simulink model "CommSysSimulink"  (R2025b)
settings: Solver=VariableStepAuto  StartTime=0.0  StopTime=1  RelTol=1e-3
model workspace (MAT data in the model file):
  iSNR = 1
  x = 0
undefined symbols (not defined in the file): alpha, filterLenSymbols, modOrder, samplesPerSymbol, SNR, symRate
libraries: commdigbbndpm3 x6, commfilt2 x2, commdigbbndam3 x2, commchan3 x1, commsink2 x1, commseqgen3 x1, commrandsrc3 x1, simulink x1, commsync2 x1
settings Model: Creator=flora  LastModifiedBy=linnh

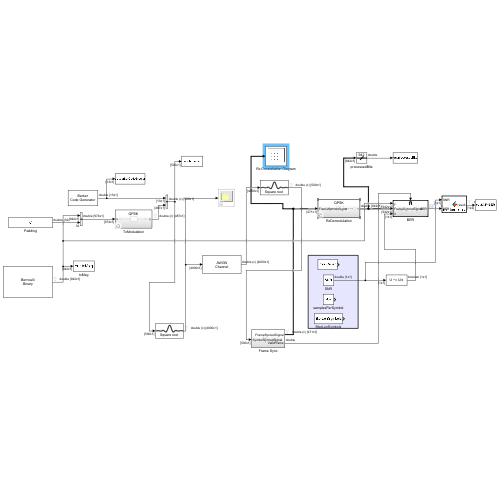
[thumbnail: Simulink's stored preview of the top-level diagram]
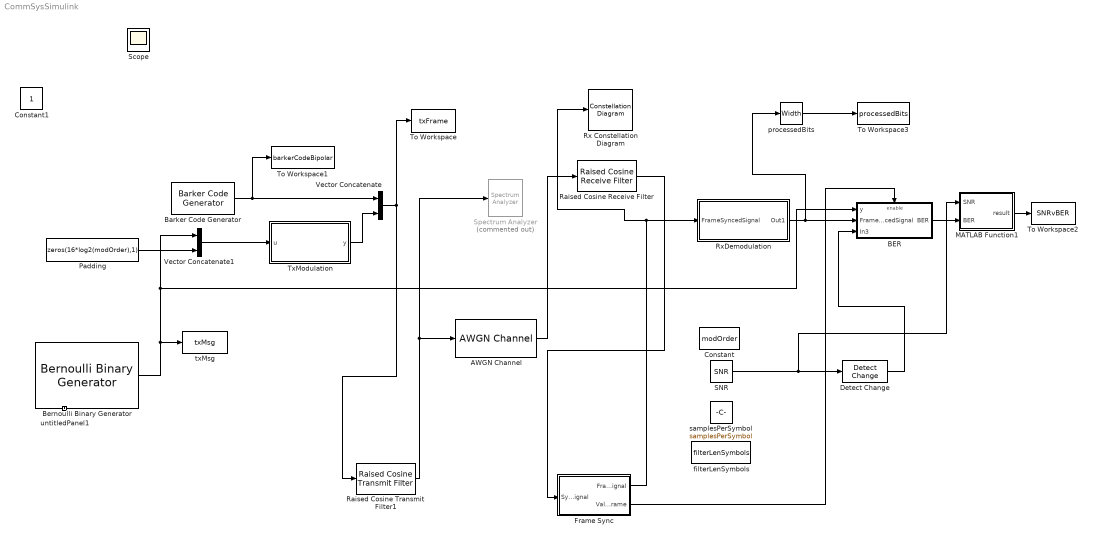
== system CommSysSimulink ==
  AWGN Channel : commchan3/AWGN Channel  LegacyMode=off  NoiseMethod="Signal to noise ratio  (Eb/No)"  noiseMode="Signal to noise ratio  (SNR)"  EbNo=SNR  EsNo=10  SNR=SNR  BitsPerSymbol=log2(modOrder)  SignalPower=1/samplesPerSymbol  SpecifySymbolPeriod=off  SamplesPerSymbol=samplesPerSymbol  SymbolPeriod=1  VarianceSource=Parameter  Variance=SNR/2  RandomStream=Global stream  Seed=67  SimulateUsing=Interpreted execution
  BER : Subsystem  TreatAsAtomicUnit=on
  Barker Code Generator : commseqgen3/Barker Code Generator  Length=7  LengthSimulink=13  SampleTime=-1  SamplesPerFrame=13  OutputDataType=double  SimulateUsing=Interpreted execution
  Bernoulli Binary Generator : commrandsrc3/Bernoulli Binary Generator  ProbabilityOfZero=0.5  SeedSource=Auto  Seed=0  SampleTime=1/(symRate*log2(modOrder))  SamplesPerFrame="(symRate  - 13 -16) * log2(modOrder)"  OutputDataType=double  SimulateUsing=Interpreted execution
  Constant : Constant  Value=modOrder
  Detect Change : simulink/Logic and Bit Operations/Detect Change  vinit=0  OutDataTypeStr=boolean
  Frame Sync : Subsystem
  MATLAB Function1 : MATLAB Function  TreatAsAtomicUnit=on
  Padding : Constant  Value=zeros(16*log2(modOrder),1)  SampleTime=-1
  Raised Cosine Receive Filter : commfilt2/Raised Cosine Receive Filter  filtType=Square root  R=alpha  filtSpan=10  N=8  downFactor=8  downOffset=0  filterGain=1  InputProcessing=Columns as channels (frame based)  RateOptions=Enforce single-rate processing  framing=Mute  checkCoeff=on  variableName=rcRxFilt  currentFiltSpan=10  D=5  inputOffset=0  sampMode=Mute  saveAsFlag=0  rateMode=Downsampling  checkGain=Normalized  launchFVT=on  roundingMode=Floor  overflowMode=off  coeffDataTypeStr=Inherit: Same word length as input  coeffMin=[]  coeffMax=[]  coeffLastDataTypeStr=Inherit: Same word length as input  accumDataTypeStr=Inherit: Same as product output  accumLastDataTypeStr=Inherit: Same as product output  outputDataTypeStr=Inherit: Same as accumulator  outputMin=[]  outputMax=[]  outputLastDataTypeStr=Inherit: Same as accumulator
  Raised Cosine Transmit Filter1 : commfilt2/Raised Cosine Transmit Filter  filtType=Square root  R=alpha  filtSpan=10  N=8  filterGain=1  InputProcessing=Columns as channels (frame based)  RateOptions=Enforce single-rate processing  framing=Mute  checkCoeff=on  variableName=rcTxFilt1  checkGain=Normalized  sampMode=Mute  saveAsFlag=0  currentFiltSpan=10  D=(10)/2  launchFVT=on  roundingMode=Floor  overflowMode=off  coeffDataTypeStr=Inherit: Same word length as input  coeffMin=[]  coeffMax=[]  coeffLastDataTypeStr=Inherit: Same word length as input  outputDataTypeStr=Inherit: Same as accumulator  outputMin=[]  outputMax=[]  outputLastDataTypeStr=Inherit: Same as accumulator
  Rx Constellation Diagram : ConstellationDiagram  WindowPosition=[320.000000,105.000000,737.000000,703.000000,]  Visible=on  ScopeFrameLocation=window  SymbolsToDisplay=100  ReferenceConstellation=BPSK  XLimits=[-2.68,2.53]  YLimits=[-2.68,2.53]  AxesLimits=[-2.68,2.53]  ShowReferenceConstellation=off
  RxDemodulation : Subsystem  Variant=on
  SNR : Constant  Value=SNR  VectorParams1D=off
  Spectrum Analyzer : SpectrumAnalyzer  Commented=on  WindowPosition=[589.000000,16.000000,654.000000,620.000000,]  ScopeFrameLocation=window  PlotAsTwoSidedSpectrum=off  Span=399999.99999999994  StartFrequency=-199999.99999999997  StopFrequency=199999.99999999997  YLimits=[-62.6319 17.8917]  ExpandToolstrip=on  SelectedToolstripTab=spectrumAnalyzerToolstrip.estimationTab
  To Workspace : ToWorkspace  VariableName=txFrame  SampleTime=-1
      settings: Save2DSignal=2-D array (concatenate along first dimension)
  To Workspace1 : ToWorkspace  VariableName=barkerCodeBipolar  SampleTime=-1
      settings: Save2DSignal=2-D array (concatenate along first dimension)
  To Workspace2 : ToWorkspace  VariableName=SNRvBER  SampleTime=-1
  To Workspace3 : ToWorkspace  VariableName=processedBits  SaveFormat=Timeseries  SampleTime=-1
  TxModulation : Subsystem  Variant=on
  Vector Concatenate : Concatenate
  Vector Concatenate1 : Concatenate
  filterLenSymbols : Constant  Value=filterLenSymbols
  processedBits : Width
  samplesPerSymbol : Constant  Value=samplesPerSymbol
  txMsg : ToWorkspace  VariableName=txMsg  SampleTime=-1
      settings: Save2DSignal=2-D array (concatenate along first dimension)
  untitledPanel1 : Subsystem  Tag=HiddenForWebPanel  IsWebBlockPanel=on
  Constant1 : Constant  IOType=siggen
  Scope : Scope
      settings: ActiveDisplayYMinimum=0.49969  ActiveDisplayYMaximum=0.49987
  wires:
  BER/1(BER) -> MATLAB Function1/2(BER)
  processedBits/1 -> To Workspace3/1
  Detect Change/1 -> BER/3(In3)
  Padding/1 -> Vector Concatenate1/2
  MATLAB Function1/1(result) -> To Workspace2/1
  TxModulation/1(y) -> Vector Concatenate/2
  Barker Code Generator/1 -> Vector Concatenate/1, To Workspace1/1
  SNR/1 -> Detect Change/1, MATLAB Function1/1(SNR)
  Bernoulli Binary Generator/1 -> txMsg/1, BER/1(y), Vector Concatenate1/1
  Vector Concatenate1/1 -> TxModulation/1(u)
  Vector Concatenate/1 -> Raised Cosine Transmit Filter1/1, To Workspace/1
  Raised Cosine Transmit Filter1/1 -> AWGN Channel/1, Spectrum Analyzer/1
  AWGN Channel/1 -> Raised Cosine Receive Filter/1
  Raised Cosine Receive Filter/1 -> Frame Sync/1(SymbolSyncedSignal)
  RxDemodulation/1(Out1) -> BER/2(FrameSyncedSignal), processedBits/1
  Frame Sync/1(FrameSyncedSignal) -> Rx Constellation Diagram/1, RxDemodulation/1(FrameSyncedSignal)
  Frame Sync/2(ValidFrame) -> BER/Enable

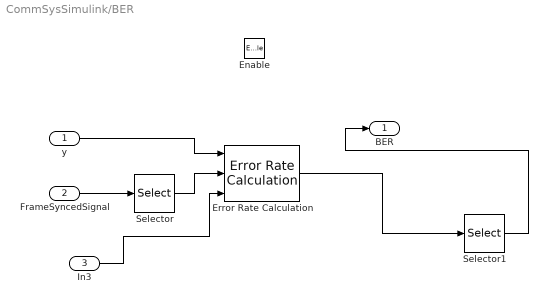
== system CommSysSimulink/BER ==
  y : Inport
  FrameSyncedSignal : Inport  Port=2
  In3 : Inport  Port=3
  Enable : EnablePort  PropagateVarSize=During execution
  Error Rate Calculation : commsink2/Error Rate Calculation  N=0  st_delay=0  cp_mode=Entire frame  subframe=[]  PMode=Port  WsName=ErrorVec  RsMode2=on  stop=off  numErr=100  maxBits=1e6
      settings: LibrarySourceBlock=|
      | commhdlsink/Error Rate
      | Calculation
  Selector : Selector  IndexOptions=Starting index (dialog)  Indices=1  OutputSizes="(symRate  - 13 -16) * log2(modOrder)"
  Selector1 : Selector  InputPortWidth=3  IndexOptions=Index vector (dialog)  Indices=1  OutputSizes=1
  BER : Outport
  wires:
  y/1 -> Error Rate Calculation/1
  Selector/1 -> Error Rate Calculation/2
  Error Rate Calculation/1 -> Selector1/1
  Selector1/1 -> BER/1
  FrameSyncedSignal/1 -> Selector/1
  In3/1 -> Error Rate Calculation/3

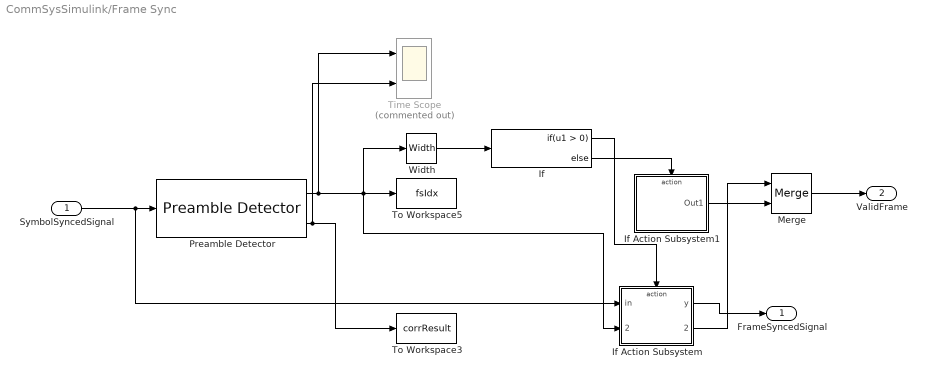
== system CommSysSimulink/Frame Sync ==
  SymbolSyncedSignal : Inport
  If : If
  If Action Subsystem : Subsystem  TreatAsAtomicUnit=on
  If Action Subsystem1 : Subsystem  TreatAsAtomicUnit=on
  Merge : Merge
  Preamble Detector : commsync2/Preamble Detector  Input=Symbol  Preamble=[-1;-1;-1;-1;-1;1;1;-1;-1;1;-1;1;-1]  Threshold=10  DetectionMetricOutput=on  Detections=First  SimulateUsing=Interpreted execution
  Time Scope : Scope  Commented=on  NumInputPorts=2
      settings: TimeUnits=Metric (based on Time Span)  Title=Preamble Detector Output  ActiveDisplayYMinimum=0  ActiveDisplayYMaximum=25  YLabel=Amplitude
  To Workspace3 : ToWorkspace  VariableName=corrResult  SaveFormat=Timeseries  SampleTime=-1
      settings: Save2DSignal=2-D array (concatenate along first dimension)
  To Workspace5 : ToWorkspace  VariableName=fsIdx  SaveFormat=Structure  SampleTime=-1
  Width : Width
  FrameSyncedSignal : Outport
  ValidFrame : Outport  Port=2
  wires:
  If Action Subsystem/1(y) -> FrameSyncedSignal/1
  Merge/1 -> ValidFrame/1
  Width/1 -> If/1
  Preamble Detector/2 -> To Workspace3/1, Time Scope/2
  If/1 -> If Action Subsystem/Action
  Preamble Detector/1 -> If Action Subsystem/2(peakIdx), To Workspace5/1, Width/1, Time Scope/1
  If Action Subsystem1/1(Out1) -> Merge/2
  If/2 -> If Action Subsystem1/Action
  SymbolSyncedSignal/1 -> Preamble Detector/1, If Action Subsystem/1(in)
  If Action Subsystem/2(ValidFrame) -> Merge/1

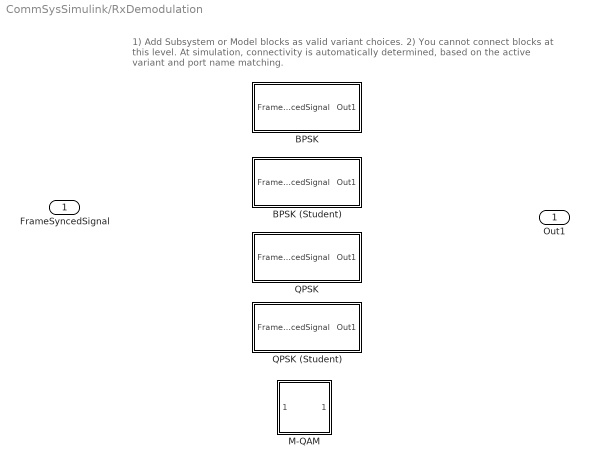
== system CommSysSimulink/RxDemodulation ==
  note: 1) Add Subsystem or Model blocks as valid variant choices.
      | 2) You cannot connect blocks at this level. At simulation, connectivity is automatically
      | determined, based on the active variant and port name matching.
  FrameSyncedSignal : Inport
  BPSK : Subsystem  VariantControl="modScheme==\"BPSK\""
  BPSK (Student) : Subsystem  VariantControl="modScheme==\"BPSK (Student)\""
  M-QAM : Subsystem  VariantControl="modScheme==\"M-QAM\""
  QPSK : Subsystem  VariantControl="modScheme==\"QPSK\""
  QPSK (Student) : Subsystem  VariantControl="modScheme==\"QPSK (Student)\""
  Out1 : Outport

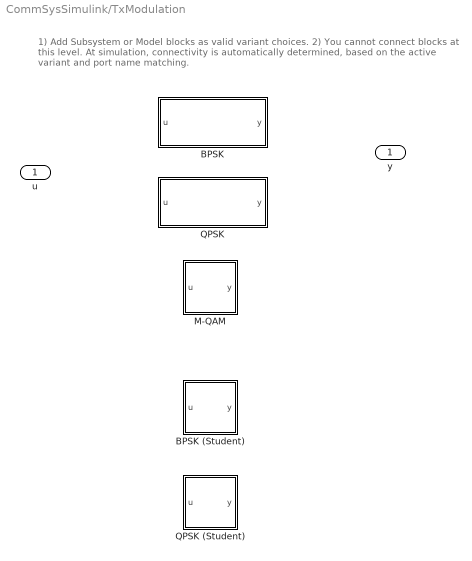
== system CommSysSimulink/TxModulation ==
  note: 1) Add Subsystem or Model blocks as valid variant choices.
      | 2) You cannot connect blocks at this level. At simulation, connectivity is automatically
      | determined, based on the active variant and port name matching.
  u : Inport
  BPSK : Subsystem  VariantControl="modScheme==\"BPSK\""
  BPSK (Student) : Subsystem  VariantControl="modScheme==\"BPSK (Student)\""
  M-QAM : Subsystem  VariantControl="modScheme==\"M-QAM\""
  QPSK : Subsystem  VariantControl="modScheme==\"QPSK\""
  QPSK (Student) : Subsystem  VariantControl="modScheme==\"QPSK (Student)\""
  y : Outport

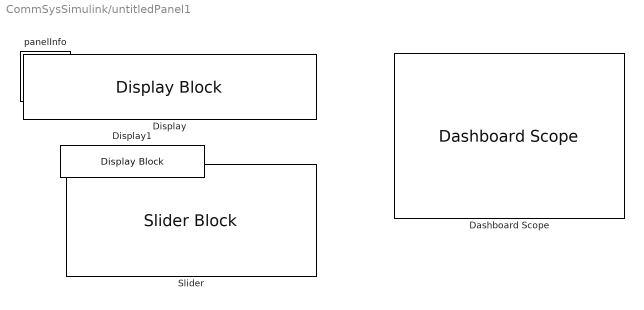
== system CommSysSimulink/untitledPanel1 ==
  Dashboard Scope : DashboardScope  Tag=HiddenForWebPanel  PanelInfo="{\"height\":234,\"left\":315,\"panelId\":\"panelId-f31e1c61-8a53-45bb-afd0-f88e0f139d22\",\"top\":52,\"type\":\"panelChild\",\"version\":\"2019b\",\"width\":354,\"zIndex\":1500004}"  Ymin=0  Ymax=1  FontColor=[0.0, 0.0, 0.0]
  Display : DisplayBlock  Tag=HiddenForWebPanel  PanelInfo="{\"height\":25,\"left\":30,\"panelId\":\"panelId-f31e1c61-8a53-45bb-afd0-f88e0f139d22\",\"top\":62,\"type\":\"panelChild\",\"version\":\"2019b\",\"width\":131,\"zIndex\":1500002}"  LabelPosition=Hide  Transparency=1  GridColor=[0.502, 0.502, 0.502]
  Display1 : DisplayBlock  Tag=HiddenForWebPanel  PanelInfo="{\"height\":30,\"left\":680,\"panelId\":\"panelId-f31e1c61-8a53-45bb-afd0-f88e0f139d22\",\"top\":36,\"type\":\"panelChild\",\"version\":\"2019b\",\"width\":135,\"zIndex\":1500008}"  LabelPosition=Hide  Transparency=1  GridColor=[0.502, 0.502, 0.502]
  Slider : SliderBlock  Tag=HiddenForWebPanel  PanelInfo="{\"height\":88,\"left\":30,\"panelId\":\"panelId-f31e1c61-8a53-45bb-afd0-f88e0f139d22\",\"top\":190,\"type\":\"panelChild\",\"version\":\"2019b\",\"width\":191,\"zIndex\":1500006}"  ScaleMin=-30  ScaleMax=30
  panelInfo : PanelWebBlock  Tag=HiddenForWebPanel  PanelInfo="{\"compacted\":false,\"height\":321,\"isActiveTab\":true,\"labels\":{\"label2052262155\":{\"deleted\":false,\"left\":32,\"settings\":{\"backgroundColor\":\"rgba(0, 0, 0, 0)\",\"bold\":false,\"font\":\"Arial\",\"fontColor\":\"black\",\"fontSize\":0.84,\"italicized\":false,\"underlined\":false},\"text\":\"SNR (dB)\",\"top\":171},\"label3800272950\":{\"deleted\":false,\"left\":25,\"settings\":{\"backgroundColor\":\"rgba(0, 0, 0, 0)\",\"bold\":false,\"font\":\"Arial\",\"fontColor\":\"black\",\"fontSize\":0.84,\"italicized\":false,\"underlined\":false},\"text\":\"Processed Bits\",\"top\":43},\"label7051701793\":{\"deleted\":false,\"left\":676,\"settings\":{\"backgroundColor\":\"rgba(0, 0, 0, 0)\",\"bold\":false,\"font\":\"Arial\",\"fontColor\":\"black\",\"fontSize\":0.84,\"italicized\":false,\"underlined\":false},\"text\":\"BER\",\"top\":14},\"label9181414523\":{\"deleted\":false,\"left\":323,\"settings\":{\"backgroundColor\":\"rgba(0, 0, 0, 0)\",\"bold\":false,\"font\":\"Arial\",\"fontColor\":\"black\",\"fontSize\":0.84,\"italicized\":false,\"underlined\":false},\"text\":\"Pulse-Shaped Symbol Stream\",\"top\":33}},\"left\":295,\"name\":\"Panel1\",\"panelId\":\"panelId-f31e1c61-8a53-45bb-afd0-f88e0f139d22\",\"tabIndex\":0,\"tabbedSetId\":\"tabbedSet4545170372\",\"top\":593,\"type\":\"panel\",\"version\":\"2019b\",\"visible\":true,\"width\":855,\"zIndex\":1500002}"  PanelSnapshot=<binary blob, 29684 chars, not shown>

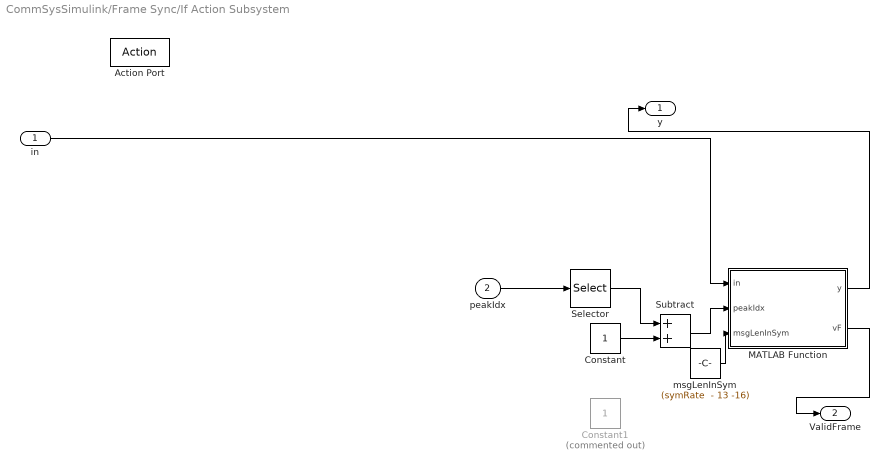
== system CommSysSimulink/Frame Sync/If Action Subsystem ==
  in : Inport
  peakIdx : Inport  Port=2
  Action Port : ActionPort  PropagateVarSize=During execution  ActionPortLabel=if(u1 > 0)
  Constant : Constant
  Constant1 : Constant  Commented=on
  MATLAB Function : MATLAB Function  TreatAsAtomicUnit=on
  Selector : Selector  InputPortWidth=1  IndexOptions=Index vector (dialog)  Indices=1  OutputSizes=1
  Subtract : Sum
  msgLenInSym : Constant  Value="(symRate  - 13 -16)"
  y : Outport
  ValidFrame : Outport  Port=2
  wires:
  Selector/1 -> Subtract/1
  in/1 -> MATLAB Function/1(in)
  Subtract/1 -> MATLAB Function/2(peakIdx)
  Constant/1 -> Subtract/2
  MATLAB Function/1(y) -> y/1
  peakIdx/1 -> Selector/1
  msgLenInSym/1 -> MATLAB Function/3(msgLenInSym)
  MATLAB Function/2(vF) -> ValidFrame/1

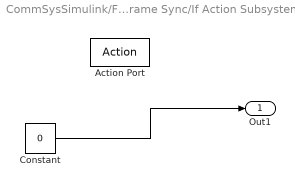
== system CommSysSimulink/Frame Sync/If Action Subsystem1 ==
  Action Port : ActionPort  ActionPortLabel=else
  Constant : Constant  Value=0
  Out1 : Outport
  wires:
  Constant/1 -> Out1/1

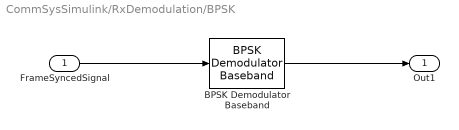
== system CommSysSimulink/RxDemodulation/BPSK ==
  FrameSyncedSignal : Inport
  BPSK Demodulator Baseband : commdigbbndpm3/BPSK Demodulator Baseband  DecType=Hard decision  VarSource=Dialog  Variance=1  Ph=0  outDtype=Inherit via internal rule  derotateFactorWordLen=16  derotateFactorDataTypeStr=Inherit: Same word length as input  derotateFactorLastDataTypeStr=Inherit: Same word length as input
  Out1 : Outport
  wires:
  FrameSyncedSignal/1 -> BPSK Demodulator Baseband/1
  BPSK Demodulator Baseband/1 -> Out1/1

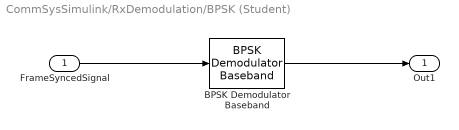
== system CommSysSimulink/RxDemodulation/BPSK (Student) ==
  FrameSyncedSignal : Inport
  BPSK Demodulator Baseband : commdigbbndpm3/BPSK Demodulator Baseband  DecType=Hard decision  VarSource=Dialog  Variance=1  Ph=0  outDtype=Inherit via internal rule  derotateFactorWordLen=16  derotateFactorDataTypeStr=Inherit: Same word length as input  derotateFactorLastDataTypeStr=Inherit: Same word length as input
  Out1 : Outport
  wires:
  FrameSyncedSignal/1 -> BPSK Demodulator Baseband/1
  BPSK Demodulator Baseband/1 -> Out1/1

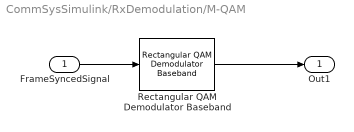
== system CommSysSimulink/RxDemodulation/M-QAM ==
  FrameSyncedSignal : Inport
  Rectangular QAM Demodulator Baseband : commdigbbndam3/Rectangular QAM Demodulator Baseband  M=modOrder  OutType=Bit  DecType=Hard decision  VarSource=Dialog  Variance=1  Dec=Gray  Mapping=[0:15]  PowType=Peak Power  MinDist=2  AvgPow=1  PeakPow=1  Ph=0  outDtype1=Inherit via internal rule  outDtype2=Inherit via internal rule  derotateFactorWordLen=16  derotateFactorDataTypeStr=Inherit: Same word length as input  derotateFactorLastDataTypeStr=Inherit: Same word length as input  denormFactorWordLen=16  denormFactorDataTypeStr=Inherit: Same word length as input  denormFactorLastDataTypeStr=Inherit: Same word length as input  prodOutWordLen=32  prodOutOverflowMode=Wrap  prodOutRoundingMode=Floor  prodOutOvFlMode=off  prodOutOvFlModeLastStrValue=off  sumWordLen=32
  Out1 : Outport
  wires:
  FrameSyncedSignal/1 -> Rectangular QAM Demodulator Baseband/1
  Rectangular QAM Demodulator Baseband/1 -> Out1/1

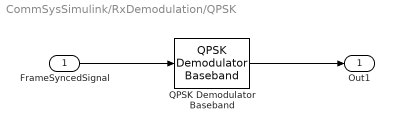
== system CommSysSimulink/RxDemodulation/QPSK ==
  FrameSyncedSignal : Inport
  QPSK Demodulator Baseband : commdigbbndpm3/QPSK Demodulator Baseband  OutType=Bit  DecType=Hard decision  VarSource=Dialog  Variance=1  Dec=Gray  Ph=pi/4  outDtype1=Inherit via internal rule  outDtype2=Inherit via internal rule  derotateFactorWordLen=16  derotateFactorDataTypeStr=Inherit: Same word length as input  derotateFactorLastDataTypeStr=Inherit: Same word length as input
      settings: LibrarySourceBlock=|
      | commhdldigbbndpm/QPSK
      | Demodulator
      | Baseband
  Out1 : Outport
  wires:
  FrameSyncedSignal/1 -> QPSK Demodulator Baseband/1
  QPSK Demodulator Baseband/1 -> Out1/1

== system CommSysSimulink/RxDemodulation/QPSK (Student) ==
  FrameSyncedSignal : Inport
  QPSK Demodulator Baseband : commdigbbndpm3/QPSK Demodulator Baseband  OutType=Bit  DecType=Hard decision  VarSource=Dialog  Variance=1  Dec=Gray  Ph=pi/4  outDtype1=Inherit via internal rule  outDtype2=Inherit via internal rule  derotateFactorWordLen=16  derotateFactorDataTypeStr=Inherit: Same word length as input  derotateFactorLastDataTypeStr=Inherit: Same word length as input
      settings: LibrarySourceBlock=|
      | commhdldigbbndpm/QPSK
      | Demodulator
      | Baseband
  Out1 : Outport
  wires:
  FrameSyncedSignal/1 -> QPSK Demodulator Baseband/1
  QPSK Demodulator Baseband/1 -> Out1/1

== system CommSysSimulink/TxModulation/BPSK ==
  u : Inport
  BPSK Modulator Baseband : commdigbbndpm3/BPSK Modulator Baseband  Ph=0  outDtype=double  outWordLen=16  outUDDataType=sfix(16)  outFracLenMode=Best precision  outFracLen=15  outDataTypeStr=double  outLastDataTypeStr=double
  y : Outport
  wires:
  u/1 -> BPSK Modulator Baseband/1
  BPSK Modulator Baseband/1 -> y/1

== system CommSysSimulink/TxModulation/BPSK (Student) ==
  u : Inport
  MATLAB Function : MATLAB Function  TreatAsAtomicUnit=on
  y : Outport
  wires:
  u/1 -> MATLAB Function/1(u)
  MATLAB Function/1(y) -> y/1

== system CommSysSimulink/TxModulation/M-QAM ==
  u : Inport
  Rectangular QAM Modulator Baseband : commdigbbndam3/Rectangular QAM Modulator Baseband  M=modOrder  InType=Bit  Enc=Gray  Mapping=[0:15]  PowType=Peak Power  MinDist=2  AvgPow=1  PeakPow=1  Ph=0  outDtype=double  outWordLen=16  outUDDataType=sfix(16)  outFracLenMode=Best precision  outFracLen=15  outDataTypeStr=double  outLastDataTypeStr=double
  y : Outport
  wires:
  u/1 -> Rectangular QAM Modulator Baseband/1
  Rectangular QAM Modulator Baseband/1 -> y/1

== system CommSysSimulink/TxModulation/QPSK ==
  u : Inport
  QPSK Modulator Baseband : commdigbbndpm3/QPSK Modulator Baseband  InType=Bit  Enc=Gray  Ph=pi/4  outDtype=double  outWordLen=16  outUDDataType=sfix(16)  outFracLenMode=Best precision  outFracLen=15  outDataTypeStr=double  outLastDataTypeStr=double
      settings: LibrarySourceBlock=|
      | commhdldigbbndpm/QPSK
      | Modulator
      | Baseband
  y : Outport
  wires:
  u/1 -> QPSK Modulator Baseband/1
  QPSK Modulator Baseband/1 -> y/1

== system CommSysSimulink/TxModulation/QPSK (Student) ==
  u : Inport
  MATLAB Function : MATLAB Function  TreatAsAtomicUnit=on
  y : Outport
  wires:
  u/1 -> MATLAB Function/1(binIn)
  MATLAB Function/1(symOut) -> y/1

== matlab function CommSysSimulink/Frame Sync/If Action Subsystem/MATLAB Function ==
  data: in input; y output size=[(symRate  - 13 -16) 1]; peakIdx input; msgLenInSym input; vF output
function [y,vF] = extractFrame(in,peakIdx, msgLenInSym)

    coder.varsize("y") % declares variables as variable-sized
   
    y = zeros(msgLenInSym, 1);

    % Boundary check
    if (peakIdx + msgLenInSym - 1) > size(in, 1)
        vF = 0;
        return 
    end

    for i = 1: msgLenInSym
        y(i,1) = in(peakIdx  + (i-1));
    end

    vF = 1;
end

== matlab function CommSysSimulink/TxModulation/BPSK (Student)/MATLAB Function ==
  data: u input; y output
function y = iBPSKmod(u)
% internal BPSKmod


coder.extrinsic("BPSKmod")
y = (0 +0i) * ones(size(u));

y = BPSKmod(u);

== matlab function CommSysSimulink/TxModulation/QPSK (Student)/MATLAB Function ==
  data: binIn input; symOut output
function symOut = QPSKmod(binIn)  % TEMPLATE SOLUTION
    %  'binIn' is a binary stream (e.g., 0100011...) with
    %  len(binIn)%log2(modOrder) = 0
    
    % Array of all odd-indexed values. (e.g., 0 0 0 1...)
    odd = binIn(1 : 2 : end);
    % Array of all even-indexed values. (e.g., 1 0 1 ...)
    even = binIn(2 : 2 : end);
    
    % In case binIn has an odd-length. 
    % (This will not haven, given len(binIn)%log2(modOrder) = 0;
    len = floor(length(binIn)/2);

    % Output
    symOut = (1/sqrt(2))*( (-1).^(even(1:len))  + (-1).^(odd(1:len))*j);

end

== matlab function CommSysSimulink/MATLAB Function1 ==
  data: SNR input; result output; BER input
function result = snr_ber_array(SNR, BER)
    % Function to return a 2D array with the given SNR and BER values
    %
    % Inputs:
    %   SNR - Signal-to-Noise Ratio (scalar)
    %   BER - Bit Error Rate (scalar)
    %
    % Output:
    %   result - 2D array containing the SNR and BER values
    
    % Ensure the inputs are scalar
    if ~isscalar(SNR) || ~isscalar(BER)
        error('Both SNR and BER must be scalar values.');
    end
    
    % Create a 2D array with SNR and BER
    result = [SNR, BER];
end
